simulink model "EV1"  (R2022b)
settings: Solver=VariableStepAuto  StartTime=0.0  StopTime=10  RelTol=1e-3
undefined symbols (not defined in the file): Ion, Lithium
libraries: spsSeriesRLCBranchLib x6, spsCurrentMeasurementLib x5, spsVoltageMeasurementLib x5, spsDiodeLib x4, spsIGBTDiodeLib x4, spsPowerLib x2, spsACVoltageSourceLib x1, spsBatteryLib x1, spsMutualInductanceLib x1, spsPWMGeneratorDCDCLib x1, spsUniversalBridgeLib x1, sps_lib x1
settings Model: Creator=Muralikrishnan  LastModifiedBy=Muralikrishnan

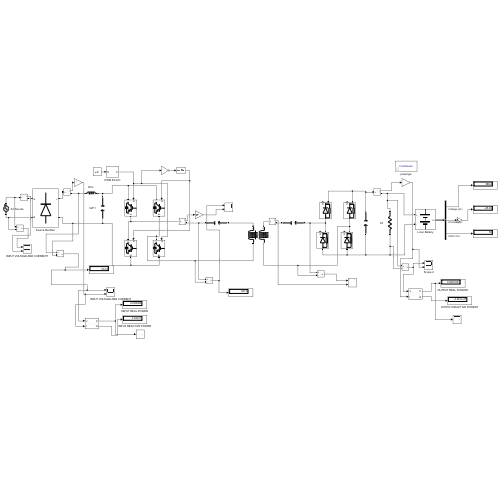
[thumbnail: Simulink's stored preview of the top-level diagram]
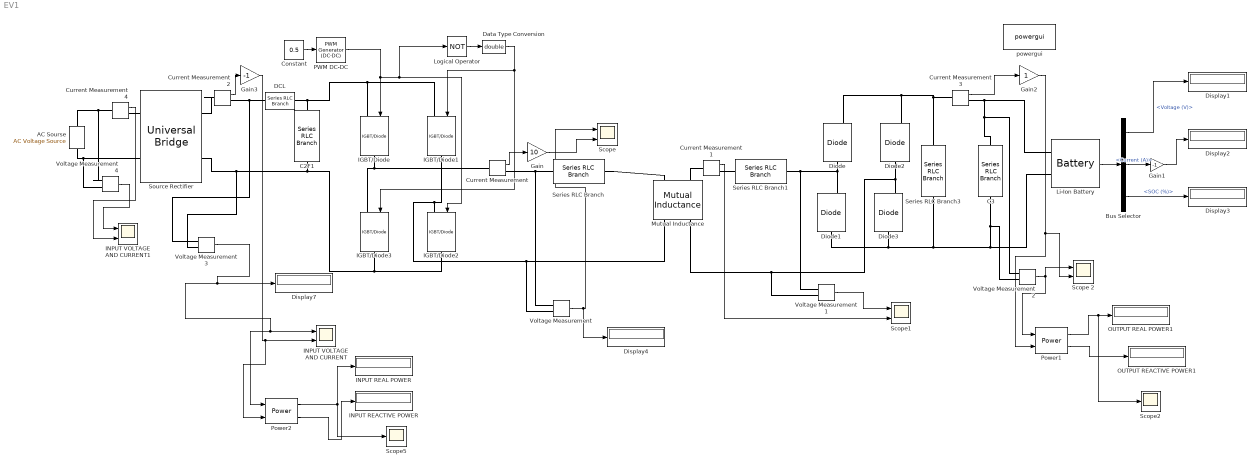
== system EV1 ==
  AC Sourse : spsACVoltageSourceLib/AC Voltage Source  Amplitude=325  Phase=0  Frequency=50  SampleTime=0  Measurements=Voltage  BusType=swing  Pref=10e3  Qref=0  Qmin=-inf  Qmax=+inf
  Bus Selector : BusSelector  OutputSignals=Voltage (V),Current (A),SOC (%)
  C2F1 : spsSeriesRLCBranchLib/Series RLC Branch  LConnTagsString=__new0  RConnTagsString=__new0  BranchType=C  Resistance=1e-6  Inductance=1e-3  SetiL0=off  InitialCurrent=0  Capacitance=300e-6  Setx0=off  InitialVoltage=0  Measurements=None
  C3 : spsSeriesRLCBranchLib/Series RLC Branch  LConnTagsString=__new0  RConnTagsString=__new0  BranchType=R  Resistance=10  Inductance=1e-3  SetiL0=off  InitialCurrent=0  Capacitance=105.74e-9  Setx0=off  InitialVoltage=0  Measurements=Branch current
  Constant : Constant  Value=0.5
  Current Measurement{,1..4} (5 alike) : spsCurrentMeasurementLib/Current Measurement  PhasorSimulation=off  OutputType=Complex  PSBequivalent=0
  DCL : spsSeriesRLCBranchLib/Series RLC Branch  LConnTagsString=__new0  RConnTagsString=__new0  BranchType=L  Resistance=0.1  Inductance=10e-3  SetiL0=off  InitialCurrent=0  Capacitance=1e-6  Setx0=off  InitialVoltage=0  Measurements=Branch current
  Data Type Conversion : DataTypeConversion  OutDataTypeStr=double  SaturateOnIntegerOverflow=off  RndMeth=Floor
  Diode{,1..3} (4 alike) : spsDiodeLib/Diode  Ron=0.001  Lon=0  Vf=0.8  IC=0  UseSnubber=0  Rs=500  Cs=250e-9  Measurements=on
  Display{1..4,7} (5 alike) : Display
  Gain : Gain  Gain=10
  Gain1 : Gain  Gain=-1
  Gain2 : Gain
  Gain3 : Gain  Gain=-1
  IGBT/Diode{,1..3} (4 alike) : spsIGBTDiodeLib/IGBT//Diode  Ron=1e-3  Rs=1e5  Cs=inf  Measurements=off
  INPUT REACTIVE POWER : Display
  INPUT REAL POWER : Display
  INPUT VOLTAGE AND CURRENT : Scope  NumInputPorts=2
  INPUT VOLTAGE AND CURRENT1 : Scope  NumInputPorts=2
  Li-Ion Battery : spsBatteryLib/Battery  BatType=Lithium-Ion  ShowTempParam=off  ThermalPreset=no  ShowAgeParam=off  NomV=360  NomQ=100  SOC=50  Batt_Tr=10  PresetModel=on  MaxQ=100  MinV=270  FullV=419.0354  Dis_rate=43.4783  R=0.036  Normal_OP=90.4348  expZone="[388.9389      4.913043]"  current=[6.5 13 32.5]  Units=Time  Tci=20  NomT=20  T2=-30  MaxQ2=4.8  FullV2=7.1  Normal_OP2=5.655  expZone2="[6.58           1]"  Rca=0.6  ti=2000  Dp=0  Neq0=0  Tsim=1e6  Ta1=25  Qeol=5.4*0.9  Reol=0.013333*1.2  Char_age=[2.3478, 3]  Dis_age=[2.3478, 10]  N1=1500  N2=10500  N3=1000  N4=1400  Ta2=45  N5=950
      settings: LibrarySourceBlock=electricdrivelib/Extra Sources/Battery
  Logical Operator : Logic  Operator=NOT  IconShape=distinctive  AllPortsSameDT=off  OutDataTypeStr=boolean
  Mutual Inductance : spsMutualInductanceLib/Mutual Inductance  LConnTagsString=a|b  RConnTagsString=A|B  TypeOfMutual=Two or three windings with equal mutual terms  NumberOfWindings=3  SelfImpedance1=[1e-3 266.16e-6]  SelfImpedance2=[1e-3 256.79e-6]  ThreeWindings=off  SelfImpedance3=[ 1.1 1.1e-03]  MutualImpedance=[0 85.46e-6]  InductanceMatrix="[1.0 0.9  0.9 ;  0.9 1.0  0.9;  0.9 0.9 1.0 ] * 1e-3"  ResistanceMatrix="[1.0 0.9  0.9 ;  0.9 1.0  0.9;  0.9 0.9 1.0 ]"  Measurements=None
      settings: LibrarySourceBlock=sps_lib/Passives/Mutual Inductance
  OUTPUT REACTIVE POWER1 : Display
  OUTPUT REAL POWER1 : Display
  PWM DC-DC : spsPWMGeneratorDCDCLib/PWM Generator (DC-DC)  Fsw=30000  Ts=0
  Power1 : spsPowerLib/Power  Freq=50  Vinit=[1, 0]  Iinit=[1, 0]  Ts=0
  Power2 : spsPowerLib/Power  Freq=50  Vinit=[1, 0]  Iinit=[1, 0]  Ts=0
  Scope : Scope  NumInputPorts=2
  Scope 2 : Scope  NumInputPorts=2
  Scope1 : Scope  NumInputPorts=2
  Scope2 : Scope
  Scope5 : Scope
  Series RLC Branch : spsSeriesRLCBranchLib/Series RLC Branch  LConnTagsString=__new0  RConnTagsString=__new0  BranchType=C  Resistance=1  Inductance=1e-3  SetiL0=off  InitialCurrent=0  Capacitance=105.74e-9  Setx0=off  InitialVoltage=0  Measurements=None
  Series RLC Branch1 : spsSeriesRLCBranchLib/Series RLC Branch  LConnTagsString=__new0  RConnTagsString=__new0  BranchType=C  Resistance=1  Inductance=1e-3  SetiL0=off  InitialCurrent=0  Capacitance=109.69e-9  Setx0=off  InitialVoltage=0  Measurements=None
  Series RLC Branch3 : spsSeriesRLCBranchLib/Series RLC Branch  LConnTagsString=__new0  RConnTagsString=__new0  BranchType=C  Resistance=1  Inductance=1e-3  SetiL0=off  InitialCurrent=0  Capacitance=300e-6  Setx0=off  InitialVoltage=0  Measurements=None
  Source Rectifier : spsUniversalBridgeLib/Universal Bridge  Arms=2  SnubberResistance=1e5  SnubberCapacitance=inf  Device=Diodes  Ron=1e-3  Lon=0  ForwardVoltages="[  0  0  ]"  ForwardVoltage=0  GTOparameters=[ 10e-6 , 20e-6 ]  IGBTparameters=[ 1e-6 , 2e-6 ]  Measurements=All voltages and currents  Measurements_2=None  converterType=Rectifier
  Voltage Measurement{,1..4} (5 alike) : spsVoltageMeasurementLib/Voltage Measurement  PhasorSimulation=off  OutputType=Complex  PSBequivalent=0
  powergui : sps_lib/powergui  Priority=1  SimulationMode=Continuous  SampleTime=1e-07  frequency=60  Iterations=50  frequencyindice=0  Pbase=100e6  ErrMax=1e-4  UnitsV=kV  UnitsW=MW  buscounter=0  FunctionMessages=off  echomessages=off  EnableUseOfTLC=off  CurrentSourceSwitches=off  DisableSnubberDevices=off  DisableRonSwitches=off  DisableVfSwitches=off  DisplayEquations=off  AutomaticDiscreteSolvers=off  SolverType=Tustin/Backward Euler (TBE)  Interpol=off  ExternalGateDelay=off  methode=off  Ts=100  x0status=blocks  SPID=on  SwTol=0  HookPort=off  NonlinearTolerance=1e-4  nMaxIteration=100  ContinueOnMaxIteration=off  RestoreLinks=warning  ResistiveCurrentMeasurement=off  Frange=[0:2:500]  Ylog=off  Xlog=on  ShowGrid=off  save=off  variable=ZData  structure=0  ZoomFFT=off  StartTime=0.0  cycles=1  DisplayStyle=1  fundamental=60  FreqAxis=off  MaxFrequency=1000  frequencyindicesteady=1  RmsSteady=1  display=off
  wires:
  Voltage Measurement/1 -> Display4/1, Scope/1
  Current Measurement1/1 -> Scope1/2
  PWM DC-DC/1 -> Logical Operator/1, IGBT/Diode2/1, IGBT/Diode/1
  Voltage Measurement3/1 -> INPUT VOLTAGE AND CURRENT/1, Power2/1, Display7/1
  Power2/2 -> INPUT REACTIVE POWER/1
  Power2/1 -> INPUT REAL POWER/1, Scope5/1
  Constant/1 -> PWM DC-DC/1
  Logical Operator/1 -> Data Type Conversion/1
  Data Type Conversion/1 -> IGBT/Diode1/1, IGBT/Diode3/1
  Li-Ion Battery/1 -> Bus Selector/1
  Bus Selector/1 -> Display1/1  "<Voltage (V)>"
  Bus Selector/3 -> Display3/1  "<SOC (%)>"
  Bus Selector/2 -> Gain1/1  "<Current (A)>"
  Voltage Measurement1/1 -> Scope1/1
  Current Measurement/1 -> Gain/1
  Gain/1 -> Scope/2
  Voltage Measurement2/1 -> Power1/1, Scope 2/1
  Power1/1 -> Scope2/1, OUTPUT REAL POWER1/1
  Power1/2 -> OUTPUT REACTIVE POWER1/1
  Gain1/1 -> Display2/1
  Current Measurement3/1 -> Gain2/1
  Gain2/1 -> Scope 2/2, Power1/2
  Current Measurement2/1 -> Gain3/1
  Gain3/1 -> Power2/2, INPUT VOLTAGE AND CURRENT/2
  Voltage Measurement4/1 -> INPUT VOLTAGE AND CURRENT1/1
  Current Measurement4/1 -> INPUT VOLTAGE AND CURRENT1/2
  connections:
  Diode3/LConn1 -- Voltage Measurement2/LConn2 -- C3/RConn1 -- Li-Ion Battery/LConn2 -- Series RLC Branch3/RConn1 -- Diode1/LConn1
  IGBT/Diode2/LConn1 -- IGBT/Diode1/RConn1 -- Voltage Measurement/LConn2 -- Mutual Inductance/RConn1
  Mutual Inductance/RConn2 -- Diode3/RConn1 -- Diode2/LConn1 -- Voltage Measurement1/LConn2
  DCL/LConn1 -- C2F1/LConn1 -- IGBT/Diode1/LConn1 -- IGBT/Diode/LConn1
  Diode/LConn1 -- Diode1/RConn1 -- Voltage Measurement1/LConn1 -- Series RLC Branch1/RConn1
  Series RLC Branch/LConn1 -- Current Measurement/RConn1 -- Voltage Measurement/LConn1
  IGBT/Diode/RConn1 -- IGBT/Diode3/LConn1 -- Current Measurement/LConn1
  IGBT/Diode2/RConn1 -- Voltage Measurement3/LConn2 -- Source Rectifier/RConn2 -- C2F1/RConn1 -- IGBT/Diode3/RConn1
  Current Measurement1/LConn1 -- Mutual Inductance/LConn2
  Current Measurement1/RConn1 -- Series RLC Branch1/LConn1
  Series RLC Branch/RConn1 -- Mutual Inductance/LConn1
  Series RLC Branch3/LConn1 -- Diode/RConn1 -- Diode2/RConn1 -- Current Measurement3/LConn1
  AC Sourse/RConn1 -- Voltage Measurement4/LConn1 -- Current Measurement4/LConn1
  Current Measurement2/LConn1 -- Source Rectifier/RConn1
  Current Measurement4/RConn1 -- Source Rectifier/LConn1
  DCL/RConn1 -- Voltage Measurement3/LConn1 -- Current Measurement2/RConn1
  AC Sourse/LConn1 -- Voltage Measurement4/LConn2 -- Source Rectifier/LConn2
  C3/LConn1 -- Li-Ion Battery/LConn1 -- Current Measurement3/RConn1 -- Voltage Measurement2/LConn1
